simulink model "DC_Motor_control_speed_Direction_Push_Button"  (R2024a)
settings: Solver=FixedStepDiscrete  StartTime=0.0  StopTime=inf  FixedStep=1e-3  RelTol=1e-3  EnableMultiTasking=on
libraries: arduinolib x6
settings Model: ExtModeTrigDuration=2  Creator=DELL  LastModifiedBy=DELL
settings SolverCC: AutoInsertRateTranBlk=on
settings OptimizationCC: EnhancedBackFolding=on  PassReuseOutputArgsAs=Individual arguments  ZeroExternalMemoryAtStartup=off  ZeroInternalMemoryAtStartup=off  MaxStackSize=64  OptimizeBlockOrder=speed  DifferentSizesBufferReuse=on  OptimizationCustomize=off  EfficientTunableParamExpr=on
settings DebuggingCC: ParameterTunabilityLossMsg=error
settings HardwareCC: ProdBitPerInt=16  ProdBitPerPointer=16  ProdBitPerSizeT=16  ProdBitPerPtrDiffT=16  ProdLargestAtomicFloat=None  ProdWordSize=8  ProdHWDeviceType=Atmel->AVR
settings SFSimCC: MATLABDynamicMemAlloc=off
settings RTWCC: Description=Embedded Coder  SystemTargetFile=ert.tlc  HardwareBoard=Arduino Uno  TemplateMakefile=ert_default_tmf  Toolchain=Arduino AVR  BuildConfiguration=Faster Runs
settings CodeAppCC: ForceParamTrailComments=on  IgnoreCustomStorageClasses=off  OperatorAnnotations=on  SimulinkDataObjDesc=on  SFDataObjDesc=on  InsertBlockDesc=on
settings ERTTargetCC: SupportContinuousTime=on  SupportVariableSizeSignals=on  ExtModeTransport=3  ExtModeStaticAlloc=on  ExtModeAutomaticAllocSize=off  ExtModeStaticAllocSize=250  ExtModeMexFile=ext_xcp  ExtModeIntrfLevel=Level2 - Open

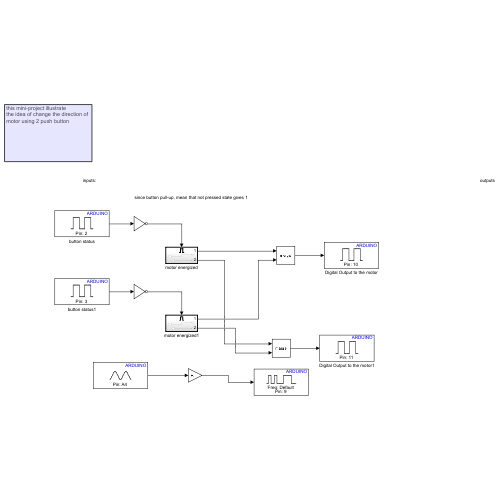
[thumbnail: Simulink's stored preview of the top-level diagram]
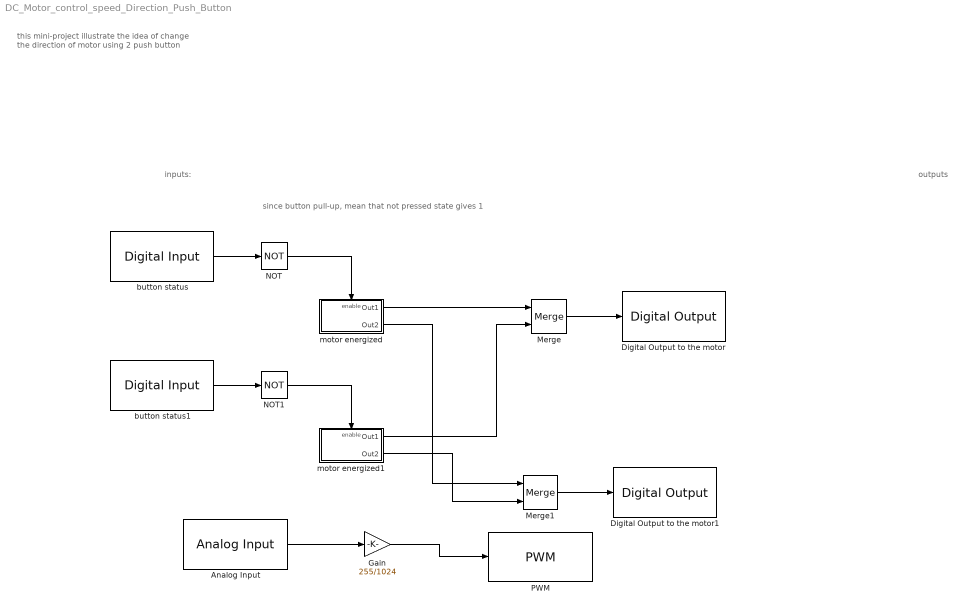
== system DC_Motor_control_speed_Direction_Push_Button ==
  note: outputs
  note: inputs:
  note: this mini-project illustrate
      | the idea of change the direction of
      | motor using 2 push button
  note: since button pull-up, mean that not pressed state gives 1
  Analog Input : arduinolib/Analog Input  pinNumber=4  ReadResultsOnly=off  ConversionTriggerSource=Software  ExternalTriggerType=uint32( 0 )  OutputDataType=uint16  EnableConversionCompleteNotify=off  EnableOuputStatus=off  SampleTime=-1  blockPlatform=arduino
  Digital Output to the motor : arduinolib/Digital Output  pinNumber=10  Direction=output  blockPlatform=arduino
  Digital Output to the motor1 : arduinolib/Digital Output  pinNumber=11  Direction=output  blockPlatform=arduino
  Gain : Gain  Gain=255/1024
  Merge : Merge
  Merge1 : Merge
  NOT : Logic  Operator=NOT  IconShape=distinctive  AllPortsSameDT=off  OutDataTypeStr=boolean
  NOT1 : Logic  Operator=NOT  IconShape=distinctive  AllPortsSameDT=off  OutDataTypeStr=boolean
  PWM : arduinolib/PWM  pinNumber=9  frequencyType=Default  desiredFrequency=490.2  achievableFrequency=490.2
  button status : arduinolib/Digital Input  pinNumber=2  mode=Input Pullup  Direction=input  SampleTime=0.1  blockPlatform=arduino
  button status1 : arduinolib/Digital Input  pinNumber=3  mode=Input Pullup  Direction=input  SampleTime=0.1  blockPlatform=arduino
  motor energized : Subsystem  TreatAsAtomicUnit=on
  motor energized1 : Subsystem  TreatAsAtomicUnit=on
  wires:
  button status/1 -> NOT/1
  button status1/1 -> NOT1/1
  Merge/1 -> Digital Output to the motor/1
  Merge1/1 -> Digital Output to the motor1/1
  NOT/1 -> motor energized/Enable
  NOT1/1 -> motor energized1/Enable
  motor energized/1(Out1) -> Merge/1
  motor energized/2(Out2) -> Merge1/1
  motor energized1/1(Out1) -> Merge/2
  motor energized1/2(Out2) -> Merge1/2
  Analog Input/1 -> Gain/1
  Gain/1 -> PWM/1

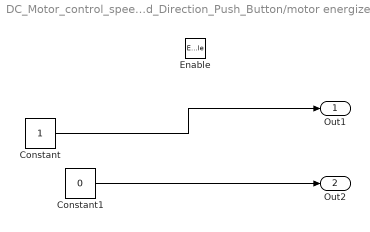
== system DC_Motor_control_speed_Direction_Push_Button/motor energized ==
  Enable : EnablePort
  Constant : Constant
  Constant1 : Constant  Value=0
  Out1 : Outport
  Out2 : Outport  Port=2
  wires:
  Constant/1 -> Out1/1
  Constant1/1 -> Out2/1

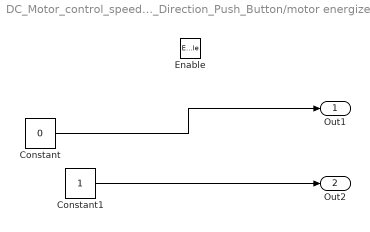
== system DC_Motor_control_speed_Direction_Push_Button/motor energized1 ==
  Enable : EnablePort
  Constant : Constant  Value=0
  Constant1 : Constant
  Out1 : Outport
  Out2 : Outport  Port=2
  wires:
  Constant1/1 -> Out2/1
  Constant/1 -> Out1/1
